simulink model "PMSMpanel_3_1502"  (Simulink 9.2)
settings: Solver=ode45  StartTime=0.0  StopTime=10  RelTol=1e-6  AbsTol=1e-8
values from neighbouring files (symbols this model uses):
  B = 0.08    [PMSMMainprog.m]
  Ba = alpha_s*J_hat - B_hat    (= 1.17)    [PMSMMainprog.m]
  Beta_1 = 113.8*pi/180    (= 1.98618468877)    [PMSMMainprog.m]
  Beta_1_time = 0    [PMSMMainprog.m]
  Beta_2 = 130*pi/180    (= 2.26892802759)    [PMSMMainprog.m]
  Beta_2_time = 2.3    [PMSMMainprog.m]
  Hcd = 1/kpcd    (= 0.0289855072464)    [PMSMMainprog.m]
  Hcq = 1/kpcq    (= 0.0116959064327)    [PMSMMainprog.m]
  i_sd0 = 0*-1.95    (= 0)    [PMSMMainprog.m]
  i_sq0 = 0*4.55    (= 0)    [PMSMMainprog.m]
  iconvlim = 6.5 * sqrt(2)    [PMSMMainprog.m]
  J = 0.0125    [PMSMMainprog.m]
  kicd = alpha_c * (Racd + R_hat)    (= 34500)    [PMSMMainprog.m]
  kicq = alpha_c * (Racq + R_hat)    (= 85500)    [PMSMMainprog.m]
  kis = alpha_s * ( Ba + B_hat)    (= 125)    [PMSMMainprog.m]
  kpcd = alpha_c * L_sd_hat    (= 34.5)    [PMSMMainprog.m]
  kpcq = alpha_c * L_sq_hat    (= 85.5)    [PMSMMainprog.m]
  kps = alpha_s  *J_hat    (= 1.25)    [PMSMMainprog.m]
  L_sd = Laa0 + Lab0 + 1.5 * Laa2    (= 0.0345)    [PMSMMainprog.m]
  L_sd_hat = 0.0345    [PMSMMainprog.m]
  L_sq = Laa0 + Lab0 - 1.5 * Laa2    (= 0.0855)    [PMSMMainprog.m]
  L_sq_hat = 0.0855    [PMSMMainprog.m]
  np = 60 * f/n_s    (= 2)    [PMSMMainprog.m]
  psi_m = 0.822    [PMSMMainprog.m]
  R = 1.33    [PMSMMainprog.m]
  Racd = alpha_c*L_sd_hat - R_hat    (= 33.17)    [PMSMMainprog.m]
  Racq = alpha_c*L_sq_hat - R_hat    (= 84.17)    [PMSMMainprog.m]
  Teref1 = 16.6    [PMSMMainprog.m]
  Teref1_time = 0.1    [PMSMMainprog.m]
  Teref2 = 4    [PMSMMainprog.m]
  Teref2_time = 2.7    [PMSMMainprog.m]
  theta_r0 = 0    [PMSMMainprog.m]
  Tstep = 4    [PMSMMainprog.m]
  Tstep_time = 1.1    [PMSMMainprog.m]
  usd0 = 0*-125    (= 0)    [PMSMMainprog.m]
  usq0 = 0*243    (= 0)    [PMSMMainprog.m]
  VconvLim = 440 * sqrt(2/3)    [PMSMMainprog.m]
  w_r0 = 0*2*pi*50/np    (= 0)    [PMSMMainprog.m]
  wrref = 1500*2*pi/60    (= 157.079632679)    [PMSMMainprog.m]
  wrref_time = 0.1    [PMSMMainprog.m]
  ws = 2*pi*50    (= 314.159265359)    [PMSMMainprog.m]    (also in PostProssPMSM.m = ones(s,1).*ws)
undefined symbols (not defined in the file or in its folder): j
settings Model: Creator=e6zebra  LastModifiedBy=Raghuram  ExtModeTrigMode=oneshot  ExtModeArmWhenConnect=off  ExtModeAutoUpdateStatusClock=off
settings SolverCC: AutoScaleAbsTol=off
settings DataIOCC: LimitDataPoints=off
settings OptimizationCC: BlockReduction=off  BooleanDataType=off  ExpressionDepthLimit=2147483647  InitFltsAndDblsToZero=on
settings DebuggingCC: SaveWithParameterizedLinksMsg=none  SignalResolutionControl=TryResolveAllWithWarning  MultiTaskDSMMsg=warning  MultiTaskCondExecSysMsg=none
settings HardwareCC: TargetUnknown=on
settings RTWCC: TemplateMakefile=grt.tmf
settings GRTTargetCC: TargetFcnLib=ansi_tfl_tmw.mat
settings ConfigComp: CovSFcnEnable=off

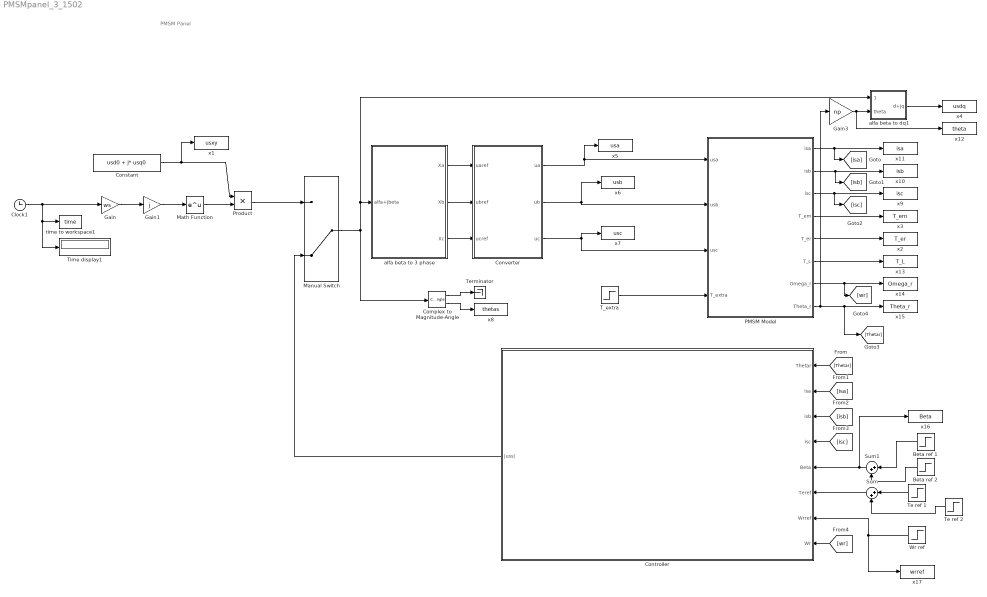
== system PMSMpanel_3_1502 ==
  note: PMSM Panel
  Beta ref 1 : Step  Time=Beta_1_time  After=Beta_1  SampleTime=0
  Beta ref 2 : Step  Time=Beta_2_time  After=Beta_2  SampleTime=0
  Clock1 : Clock
  Complex to Magnitude-Angle : ComplexToMagnitudeAngle
  Constant : Constant  Value=usd0 + j* usq0
  Controller : Subsystem
  Converter : Subsystem
  Gain : Gain  Gain=ws
  Gain1 : Gain  Gain=j
  Gain3 : Gain  Gain=np
  Manual Switch : ManualSwitch  CurrentSetting=0
  Math Function : Math  SaturateOnIntegerOverflow=on
  PMSM Model : Subsystem
  Product : Product
  Sum : Sum  Inputs=|++
  Sum1 : Sum  Inputs=|++
  T_extra : Step  Time=Tstep_time  After=Tstep  SampleTime=0
  Te ref 1 : Step  Time=Teref1_time  After=Teref1  SampleTime=0
  Te ref 2 : Step  Time=Teref2_time  After=Teref2  SampleTime=0
  Terminator : Terminator
  Time display1 : Display
  Wr ref : Step  Time=wrref_time  After=wrref  SampleTime=0
  alfa beta to 3 phase : Subsystem
  alfa beta to dq1 : Subsystem
  time to workspace1 : ToWorkspace  VariableName=time  SampleTime=-1
  x1 : ToWorkspace  VariableName=usxy  SampleTime=-1
  x10 : ToWorkspace  VariableName=isb  SampleTime=-1
  x11 : ToWorkspace  VariableName=isa  SampleTime=-1
  x12 : ToWorkspace  VariableName=theta  SampleTime=-1
  x13 : ToWorkspace  VariableName=T_L  SampleTime=-1
  x14 : ToWorkspace  VariableName=Omega_r  SampleTime=-1
  x15 : ToWorkspace  VariableName=Theta_r  SampleTime=-1
  x16 : ToWorkspace  VariableName=Beta  SampleTime=-1
  x17 : ToWorkspace  VariableName=wrref  SampleTime=-1
  x2 : ToWorkspace  VariableName=T_er  SampleTime=-1
  x3 : ToWorkspace  VariableName=T_em  SampleTime=-1
  x4 : ToWorkspace  VariableName=usdq  SampleTime=-1
  x5 : ToWorkspace  VariableName=usa  SampleTime=-1
  x6 : ToWorkspace  VariableName=usb  SampleTime=-1
  x7 : ToWorkspace  VariableName=usc  SampleTime=-1
  x8 : ToWorkspace  VariableName=thetas  SampleTime=-1
  x9 : ToWorkspace  VariableName=isc  SampleTime=-1
  wires:
  PMSM Model/3(isc) -> [isc], x9/1
  PMSM Model/1(isa) -> [isa], x11/1
  PMSM Model/2(isb) -> [isb], x10/1
  Converter/1(ua) -> x5/1, PMSM Model/1(usa)
  Converter/2(ub) -> x6/1, PMSM Model/2(usb)
  Converter/3(uc) -> PMSM Model/3(usc), x7/1
  T_extra/1 -> PMSM Model/4(T_extra)
  PMSM Model/6(T_L) -> x13/1
  PMSM Model/7(Omega_r) -> [wr], x14/1
  PMSM Model/5(T_er) -> x2/1
  PMSM Model/4(T_em) -> x3/1
  Gain1/1 -> Math Function/1
  Gain/1 -> Gain1/1
  Math Function/1 -> Product/2
  Constant/1 -> Product/1, x1/1
  Clock1/1 -> Time display1/1, time to workspace1/1, Gain/1
  Manual Switch/1 -> Complex to Magnitude-Angle/1, alfa beta to dq1/1(alfa+jbeta), alfa beta to 3 phase/1(alfa+jbeta)
  alfa beta to 3 phase/1(Xa) -> Converter/1(uaref)
  alfa beta to 3 phase/2(Xb) -> Converter/2(ubref)
  alfa beta to 3 phase/3(Xc) -> Converter/3(ucref)
  alfa beta to dq1/1(d+jq) -> x4/1
  Complex to Magnitude-Angle/1 -> Terminator/1
  Complex to Magnitude-Angle/2 -> x8/1
  PMSM Model/8(Theta_r) -> [Thetar], x15/1, Gain3/1
  Gain3/1 -> x12/1, alfa beta to dq1/2(theta)
  Product/1 -> Manual Switch/1
  [Thetar] -> Controller/1(Thetar)
  [isa] -> Controller/2(isa)
  [isb] -> Controller/3(isb)
  [isc] -> Controller/4(isc)
  Wr ref/1 -> Controller/7(Wrref), x17/1
  Controller/1(|uss|) -> Manual Switch/2
  [wr] -> Controller/8(Wr)
  Te ref 2/1 -> Sum/2
  Te ref 1/1 -> Sum/1
  Sum/1 -> Controller/6(Teref)
  Beta ref 1/1 -> Sum1/1
  Beta ref 2/1 -> Sum1/2
  Sum1/1 -> Controller/5(Beta), x16/1

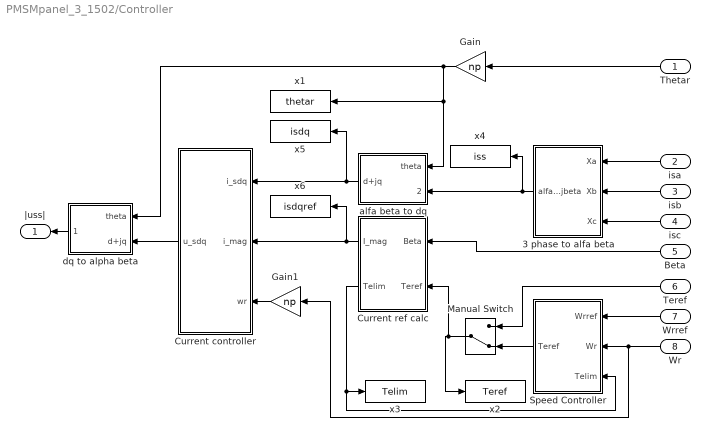
== system PMSMpanel_3_1502/Controller ==
  Thetar : Inport
  isa : Inport  Port=2
  isb : Inport  Port=3
  isc : Inport  Port=4
  Beta : Inport  Port=5
  Teref : Inport  Port=6
  Wrref : Inport  Port=7
  Wr : Inport  Port=8
  3 phase to alfa beta : Subsystem
  Current controller : Subsystem
  Current ref calc : Subsystem
  Gain : Gain  Gain=np
  Gain1 : Gain  Gain=np
  Manual Switch : ManualSwitch  CurrentSetting=0
  Speed Controller : Subsystem
  alfa beta to dq : Subsystem
  dq to alpha beta : Subsystem
  x1 : ToWorkspace  VariableName=thetar  SampleTime=-1
  x2 : ToWorkspace  VariableName=Teref  SampleTime=-1
  x3 : ToWorkspace  VariableName=Telim  SampleTime=-1
  x4 : ToWorkspace  VariableName=iss  SampleTime=-1
  x5 : ToWorkspace  VariableName=isdq  SampleTime=-1
  x6 : ToWorkspace  VariableName=isdqref  SampleTime=-1
  |uss| : Outport
  wires:
  isa/1 -> 3 phase to alfa beta/1(Xa)
  isb/1 -> 3 phase to alfa beta/2(Xb)
  isc/1 -> 3 phase to alfa beta/3(Xc)
  Thetar/1 -> Gain/1
  3 phase to alfa beta/1(alfa+jbeta) -> alfa beta to dq/2(alfa+jbeta), x4/1
  Gain/1 -> x1/1, alfa beta to dq/1(theta), dq to alpha beta/1(theta)
  dq to alpha beta/1(alfa+jbeta) -> |uss|/1
  Wrref/1 -> Speed Controller/1(Wrref)
  Wr/1 -> Gain1/1, Speed Controller/2(Wr)
  Teref/1 -> Manual Switch/1
  Speed Controller/1(Teref) -> Manual Switch/2
  Beta/1 -> Current ref calc/1(Beta)
  Manual Switch/1 -> Current ref calc/2(Teref), x2/1
  Gain1/1 -> Current controller/3(wr)
  Current ref calc/2(Telim) -> x3/1, Speed Controller/3(Telim)
  alfa beta to dq/1(d+jq) -> x5/1, Current controller/1(i_sdq)
  Current controller/1(u_sdq) -> dq to alpha beta/2(d+jq)
  Current ref calc/1(I_mag) -> Current controller/2(i_mag), x6/1

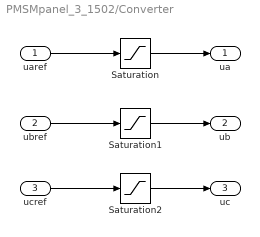
== system PMSMpanel_3_1502/Converter ==
  uaref : Inport
  ubref : Inport  Port=2
  ucref : Inport  Port=3
  Saturation : Saturate  UpperLimit=VconvLim  LowerLimit=-VconvLim
  Saturation1 : Saturate  UpperLimit=VconvLim  LowerLimit=-VconvLim
  Saturation2 : Saturate  UpperLimit=VconvLim  LowerLimit=-VconvLim
  ua : Outport
  ub : Outport  Port=2
  uc : Outport  Port=3
  wires:
  Saturation2/1 -> uc/1
  Saturation1/1 -> ub/1
  Saturation/1 -> ua/1
  uaref/1 -> Saturation/1
  ubref/1 -> Saturation1/1
  ucref/1 -> Saturation2/1

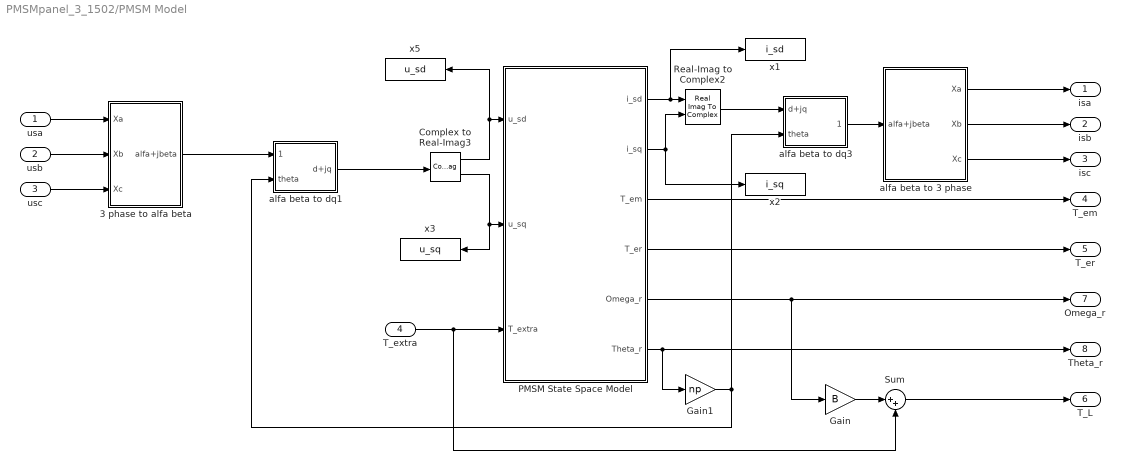
== system PMSMpanel_3_1502/PMSM Model ==
  usa : Inport
  usb : Inport  Port=2
  usc : Inport  Port=3
  T_extra : Inport  Port=4
  3 phase to alfa beta : Subsystem
  Complex to Real-Imag3 : ComplexToRealImag
  Gain : Gain  Gain=B
  Gain1 : Gain  Gain=np
  PMSM State Space Model : Subsystem
  Real-Imag to Complex2 : RealImagToComplex
  Sum : Sum  Inputs=|++
  alfa beta to 3 phase : Subsystem
  alfa beta to dq1 : Subsystem
  alfa beta to dq3 : Subsystem
  x1 : ToWorkspace  VariableName=i_sd  SampleTime=-1
  x2 : ToWorkspace  VariableName=i_sq  SampleTime=-1
  x3 : ToWorkspace  VariableName=u_sq  SampleTime=-1
  x5 : ToWorkspace  VariableName=u_sd  SampleTime=-1
  isa : Outport
  isb : Outport  Port=2
  isc : Outport  Port=3
  T_em : Outport  Port=4
  T_er : Outport  Port=5
  T_L : Outport  Port=6
  Omega_r : Outport  Port=7
  Theta_r : Outport  Port=8
  wires:
  3 phase to alfa beta/1(alfa+jbeta) -> alfa beta to dq1/1(alfa+jbeta)
  alfa beta to dq1/1(d+jq) -> Complex to Real-Imag3/1
  usb/1 -> 3 phase to alfa beta/2(Xb)
  usc/1 -> 3 phase to alfa beta/3(Xc)
  usa/1 -> 3 phase to alfa beta/1(Xa)
  alfa beta to 3 phase/1(Xa) -> isa/1
  alfa beta to 3 phase/2(Xb) -> isb/1
  alfa beta to 3 phase/3(Xc) -> isc/1
  Real-Imag to Complex2/1 -> alfa beta to dq3/1(d+jq)
  alfa beta to dq3/1(alfa+jbeta) -> alfa beta to 3 phase/1(alfa+jbeta)
  T_extra/1 -> PMSM State Space Model/3(T_extra), Sum/2
  Gain/1 -> Sum/1
  Sum/1 -> T_L/1
  Gain1/1 -> alfa beta to dq3/2(theta), alfa beta to dq1/2(theta)
  Complex to Real-Imag3/2 -> x3/1, PMSM State Space Model/2(u_sq)
  Complex to Real-Imag3/1 -> PMSM State Space Model/1(u_sd), x5/1
  PMSM State Space Model/1(i_sd) -> x1/1, Real-Imag to Complex2/1
  PMSM State Space Model/2(i_sq) -> x2/1, Real-Imag to Complex2/2
  PMSM State Space Model/6(Theta_r) -> Gain1/1, Theta_r/1
  PMSM State Space Model/5(Omega_r) -> Gain/1, Omega_r/1
  PMSM State Space Model/4(T_er) -> T_er/1
  PMSM State Space Model/3(T_em) -> T_em/1

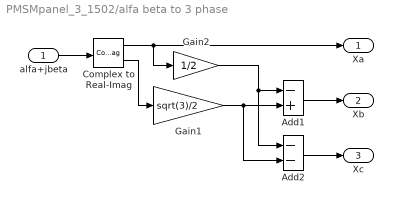
== system PMSMpanel_3_1502/alfa beta to 3 phase ==
  alfa+jbeta : Inport
  Add1 : Sum  Inputs=-+
  Add2 : Sum  Inputs=--
  Complex to Real-Imag : ComplexToRealImag
  Gain1 : Gain  Gain=sqrt(3)/2
  Gain2 : Gain  Gain=1/2
  Xa : Outport
  Xb : Outport  Port=2
  Xc : Outport  Port=3
  wires:
  alfa+jbeta/1 -> Complex to Real-Imag/1
  Complex to Real-Imag/1 -> Xa/1, Gain2/1
  Add2/1 -> Xc/1
  Add1/1 -> Xb/1
  Complex to Real-Imag/2 -> Gain1/1
  Gain1/1 -> Add1/2, Add2/2
  Gain2/1 -> Add1/1, Add2/1

== system PMSMpanel_3_1502/alfa beta to dq1 ==
  alfa+jbeta : Inport
  theta : Inport  Port=2
  Gain : Gain  Gain=-j  SaturateOnIntegerOverflow=on  OutDataTypeStr=Inherit: Same as input  ParamDataTypeStr=Inherit: Same as input
  Math Function : Math  SaturateOnIntegerOverflow=on
  Product : Product  SaturateOnIntegerOverflow=on  OutDataTypeStr=Inherit: Same as first input
  d+jq : Outport
  wires:
  theta/1 -> Gain/1
  Gain/1 -> Math Function/1
  Math Function/1 -> Product/2
  alfa+jbeta/1 -> Product/1
  Product/1 -> d+jq/1

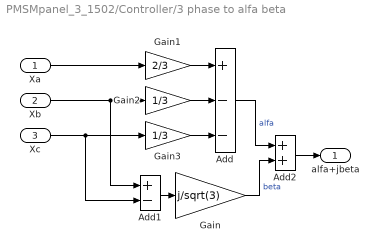
== system PMSMpanel_3_1502/Controller/3 phase to alfa beta ==
  Xa : Inport
  Xb : Inport  Port=2
  Xc : Inport  Port=3
  Add : Sum  Inputs=+--
  Add1 : Sum  Inputs=+-
  Add2 : Sum
  Gain : Gain  Gain=j/sqrt(3)
  Gain1 : Gain  Gain=2/3
  Gain2 : Gain  Gain=1/3
  Gain3 : Gain  Gain=1/3
  alfa+jbeta : Outport
  wires:
  Add1/1 -> Gain/1
  Add2/1 -> alfa+jbeta/1
  Gain/1 -> Add2/2  "beta"
  Add/1 -> Add2/1  "alfa"
  Gain3/1 -> Add/3
  Gain2/1 -> Add/2
  Gain1/1 -> Add/1
  Xa/1 -> Gain1/1
  Xb/1 -> Gain2/1, Add1/1
  Xc/1 -> Gain3/1, Add1/2

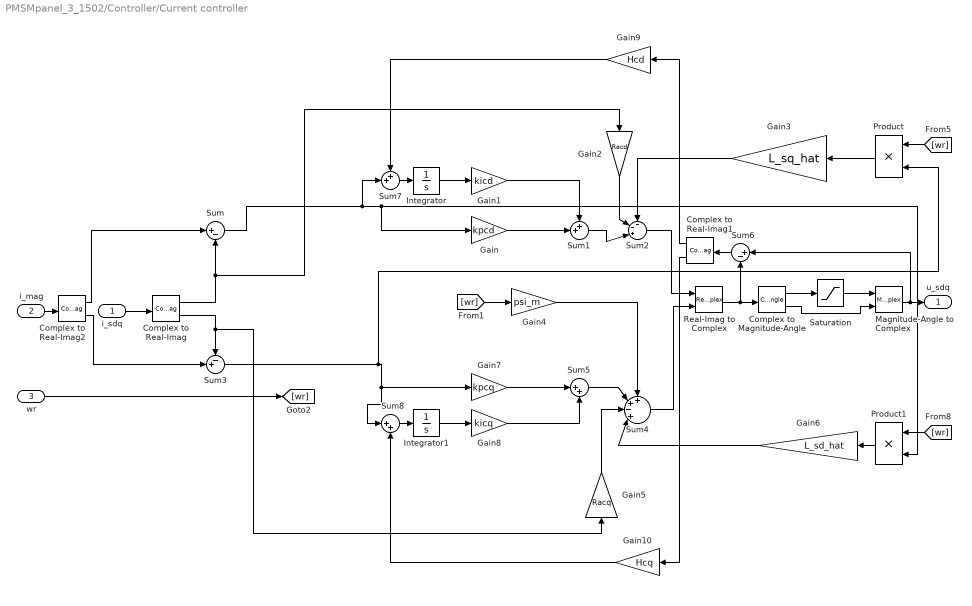
== system PMSMpanel_3_1502/Controller/Current controller ==
  i_sdq : Inport
  i_mag : Inport  Port=2
  wr : Inport  Port=3
  Complex to Magnitude-Angle : ComplexToMagnitudeAngle
  Complex to Real-Imag : ComplexToRealImag
  Complex to Real-Imag1 : ComplexToRealImag
  Complex to Real-Imag2 : ComplexToRealImag
  Gain : Gain  Gain=kpcd
  Gain1 : Gain  Gain=kicd
  Gain10 : Gain  Gain=Hcq
  Gain2 : Gain  Gain=Racd
  Gain3 : Gain  Gain=L_sq_hat
  Gain4 : Gain  Gain=psi_m
  Gain5 : Gain  Gain=Racq
  Gain6 : Gain  Gain=L_sd_hat
  Gain7 : Gain  Gain=kpcq
  Gain8 : Gain  Gain=kicq
  Gain9 : Gain  Gain=Hcd
  Integrator : Integrator  InitialCondition=i_sd0
  Integrator1 : Integrator  InitialCondition=i_sq0
  Magnitude-Angle to Complex : MagnitudeAngleToComplex
  Product : Product
  Product1 : Product
  Real-Imag to Complex : RealImagToComplex
  Saturation : Saturate  UpperLimit=VconvLim  LowerLimit=-VconvLim
  Sum : Sum  Inputs=|+-
  Sum1 : Sum  Inputs=++|
  Sum2 : Sum  Inputs=--+|
  Sum3 : Sum  Inputs=-+|
  Sum4 : Sum  Inputs=++-+|
  Sum5 : Sum  Inputs=|++
  Sum6 : Sum  Inputs=|+-
  Sum7 : Sum  Inputs=++|
  Sum8 : Sum  Inputs=|++
  u_sdq : Outport
  wires:
  wr/1 -> [wr]
  Gain/1 -> Sum1/2
  Gain1/1 -> Sum1/1
  Integrator/1 -> Gain1/1
  Sum1/1 -> Sum2/3
  Complex to Real-Imag/1 -> Gain2/1, Sum/2
  Gain2/1 -> Sum2/2
  [wr] -> Product/1
  Sum3/1 -> Product/2, Sum8/1, Gain7/1
  Product/1 -> Gain3/1
  Gain3/1 -> Sum2/1
  Sum2/1 -> Real-Imag to Complex/1
  [wr] -> Gain4/1
  i_sdq/1 -> Complex to Real-Imag/1
  Gain4/1 -> Sum4/1
  Complex to Real-Imag/2 -> Gain5/1, Sum3/1
  Gain5/1 -> Sum4/3
  Product1/1 -> Gain6/1
  Sum/1 -> Product1/2, Gain/1, Sum7/2
  [wr] -> Product1/1
  Gain6/1 -> Sum4/4
  Sum4/1 -> Real-Imag to Complex/2
  Integrator1/1 -> Gain8/1
  Gain8/1 -> Sum5/2
  Gain7/1 -> Sum5/1
  Sum5/1 -> Sum4/2
  Real-Imag to Complex/1 -> Sum6/2, Complex to Magnitude-Angle/1
  Complex to Magnitude-Angle/1 -> Saturation/1
  Saturation/1 -> Magnitude-Angle to Complex/1
  Complex to Magnitude-Angle/2 -> Magnitude-Angle to Complex/2
  Magnitude-Angle to Complex/1 -> Sum6/1, u_sdq/1
  Sum6/1 -> Complex to Real-Imag1/1
  Complex to Real-Imag1/2 -> Gain10/1
  Complex to Real-Imag1/1 -> Gain9/1
  Sum7/1 -> Integrator/1
  Gain9/1 -> Sum7/1
  Sum8/1 -> Integrator1/1
  Gain10/1 -> Sum8/2
  i_mag/1 -> Complex to Real-Imag2/1
  Complex to Real-Imag2/1 -> Sum/1
  Complex to Real-Imag2/2 -> Sum3/2

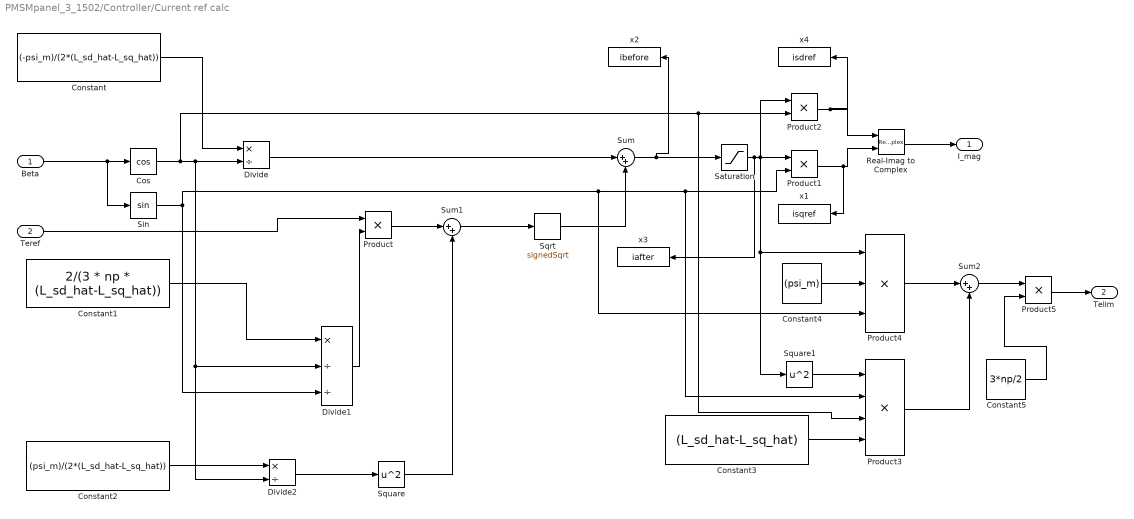
== system PMSMpanel_3_1502/Controller/Current ref calc ==
  Beta : Inport
  Teref : Inport  Port=2
  Constant : Constant  Value=(-psi_m)/(2*(L_sd_hat-L_sq_hat))
  Constant1 : Constant  Value=2/(3 * np * (L_sd_hat-L_sq_hat))
  Constant2 : Constant  Value=(psi_m)/(2*(L_sd_hat-L_sq_hat))
  Constant3 : Constant  Value=(L_sd_hat-L_sq_hat)
  Constant4 : Constant  Value=(psi_m)
  Constant5 : Constant  Value=3*np/2
  Cos : Trigonometry  Operator=cos
  Divide : Product  Inputs=*/
  Divide1 : Product  Inputs=*//
  Divide2 : Product  Inputs=*/
  Product{,1..2,5} (4 alike) : Product
  Product3 : Product  Inputs=4
  Product4 : Product  Inputs=3
  Real-Imag to Complex : RealImagToComplex
  Saturation : Saturate  UpperLimit=iconvlim  LowerLimit=-iconvlim
  Sin : Trigonometry
  Sqrt : Sqrt  Operator=signedSqrt  SaturateOnIntegerOverflow=on
  Square : Math  Operator=square  SaturateOnIntegerOverflow=on
  Square1 : Math  Operator=square  SaturateOnIntegerOverflow=on
  Sum : Sum  Inputs=|++
  Sum1 : Sum  Inputs=|++
  Sum2 : Sum  Inputs=|++
  x1 : ToWorkspace  VariableName=isqref  SampleTime=-1
  x2 : ToWorkspace  VariableName=ibefore  SampleTime=-1
  x3 : ToWorkspace  VariableName=iafter  SampleTime=-1
  x4 : ToWorkspace  VariableName=isdref  SampleTime=-1
  I_mag : Outport  VectorParamsAs1DForOutWhenUnconnected=on
  Telim : Outport  Port=2  VectorParamsAs1DForOutWhenUnconnected=on
  wires:
  Beta/1 -> Sin/1, Cos/1
  Cos/1 -> Product3/3, Product2/2, Divide2/2, Divide1/2, Divide/2
  Constant/1 -> Divide/1
  Divide/1 -> Sum/1
  Constant1/1 -> Divide1/1
  Sin/1 -> Divide1/3, Product4/3, Product3/2, Product1/2
  Divide1/1 -> Product/2
  Teref/1 -> Product/1
  Product/1 -> Sum1/1
  Constant2/1 -> Divide2/1
  Divide2/1 -> Square/1
  Square/1 -> Sum1/2
  Sum1/1 -> Sqrt/1
  Sqrt/1 -> Sum/2
  Saturation/1 -> x3/1, Product4/1, Square1/1, Product2/1, Product1/1
  Product2/1 -> x4/1, Real-Imag to Complex/1
  Product1/1 -> x1/1, Real-Imag to Complex/2
  Real-Imag to Complex/1 -> I_mag/1
  Square1/1 -> Product3/1
  Constant3/1 -> Product3/4
  Constant4/1 -> Product4/2
  Product4/1 -> Sum2/1
  Product3/1 -> Sum2/2
  Sum2/1 -> Product5/1
  Constant5/1 -> Product5/2
  Product5/1 -> Telim/1
  Sum/1 -> x2/1, Saturation/1

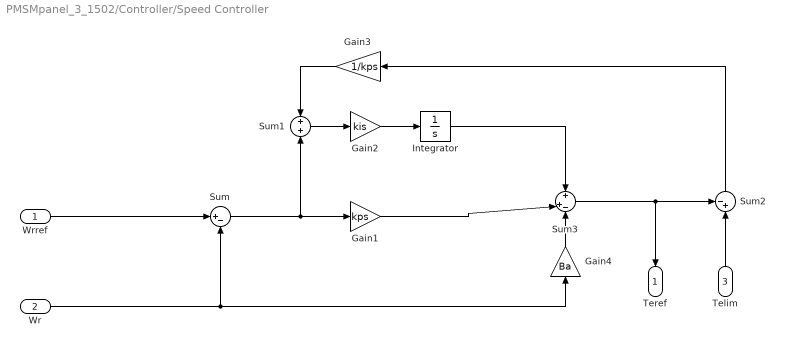
== system PMSMpanel_3_1502/Controller/Speed Controller ==
  Wrref : Inport
  Wr : Inport  Port=2
  Telim : Inport  Port=3
  Gain1 : Gain  Gain=kps
  Gain2 : Gain  Gain=kis
  Gain3 : Gain  Gain=1/kps
  Gain4 : Gain  Gain=Ba
  Integrator : Integrator
  Sum : Sum  Inputs=|+-
  Sum1 : Sum  Inputs=+|+
  Sum2 : Sum  Inputs=-+|
  Sum3 : Sum  Inputs=+|+-
  Teref : Outport
  wires:
  Sum1/1 -> Gain2/1
  Gain2/1 -> Integrator/1
  Gain3/1 -> Sum1/1
  Integrator/1 -> Sum3/1
  Sum/1 -> Gain1/1, Sum1/2
  Wrref/1 -> Sum/1
  Wr/1 -> Sum/2, Gain4/1
  Gain4/1 -> Sum3/3
  Gain1/1 -> Sum3/2
  Sum3/1 -> Teref/1, Sum2/1
  Telim/1 -> Sum2/2
  Sum2/1 -> Gain3/1

== system PMSMpanel_3_1502/Controller/alfa beta to dq ==
  theta : Inport
  alfa+jbeta : Inport  Port=2
  Gain : Gain  Gain=-j  SaturateOnIntegerOverflow=on  OutDataTypeStr=Inherit: Same as input  ParamDataTypeStr=Inherit: Same as input
  Math Function : Math  SaturateOnIntegerOverflow=on
  Product : Product  SaturateOnIntegerOverflow=on  OutDataTypeStr=Inherit: Same as first input
  d+jq : Outport
  wires:
  theta/1 -> Gain/1
  Gain/1 -> Math Function/1
  Math Function/1 -> Product/2
  alfa+jbeta/1 -> Product/1
  Product/1 -> d+jq/1

== system PMSMpanel_3_1502/Controller/dq to alpha beta ==
  theta : Inport
  d+jq : Inport  Port=2
  Gain : Gain  Gain=j  SaturateOnIntegerOverflow=on  OutDataTypeStr=Inherit: Same as input  ParamDataTypeStr=Inherit: Same as input
  Math Function : Math  SaturateOnIntegerOverflow=on
  Product : Product  SaturateOnIntegerOverflow=on  OutDataTypeStr=Inherit: Same as first input
  alfa+jbeta : Outport
  wires:
  Product/1 -> alfa+jbeta/1
  d+jq/1 -> Product/1
  Math Function/1 -> Product/2
  Gain/1 -> Math Function/1
  theta/1 -> Gain/1

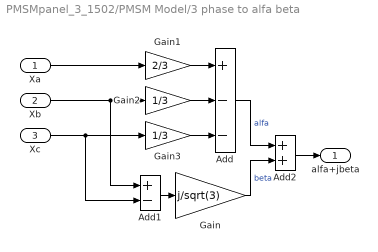
== system PMSMpanel_3_1502/PMSM Model/3 phase to alfa beta ==
  Xa : Inport
  Xb : Inport  Port=2
  Xc : Inport  Port=3
  Add : Sum  Inputs=+--
  Add1 : Sum  Inputs=+-
  Add2 : Sum
  Gain : Gain  Gain=j/sqrt(3)
  Gain1 : Gain  Gain=2/3
  Gain2 : Gain  Gain=1/3
  Gain3 : Gain  Gain=1/3
  alfa+jbeta : Outport
  wires:
  Add1/1 -> Gain/1
  Add2/1 -> alfa+jbeta/1
  Gain/1 -> Add2/2  "beta"
  Add/1 -> Add2/1  "alfa"
  Gain3/1 -> Add/3
  Gain2/1 -> Add/2
  Gain1/1 -> Add/1
  Xa/1 -> Gain1/1
  Xb/1 -> Gain2/1, Add1/1
  Xc/1 -> Gain3/1, Add1/2

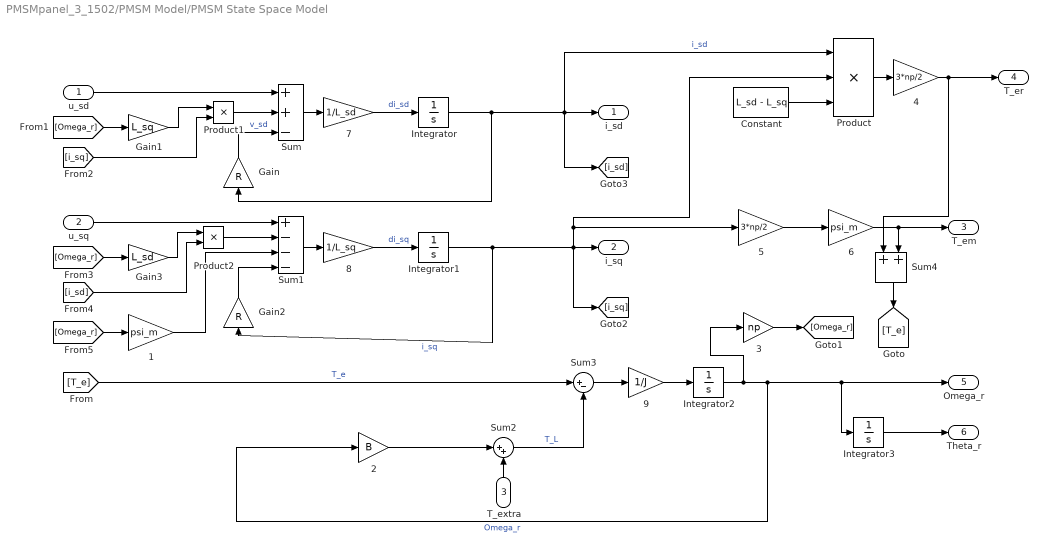
== system PMSMpanel_3_1502/PMSM Model/PMSM State Space Model ==
  u_sd : Inport
  u_sq : Inport  Port=2
  T_extra : Inport  Port=3
  "  1" : Gain  Gain=psi_m
  "  2" : Gain  Gain=B
  "  3" : Gain  Gain=np
  "  4" : Gain  Gain=3*np/2
  "  5" : Gain  Gain=3*np/2
  "  6" : Gain  Gain=psi_m
  "  7" : Gain  Gain=1/L_sd
  "  8" : Gain  Gain=1/L_sq
  "  9" : Gain  Gain=1/J
  Constant : Constant  Value=L_sd - L_sq
  Gain : Gain  Gain=R
  Gain1 : Gain  Gain=L_sq
  Gain2 : Gain  Gain=R
  Gain3 : Gain  Gain=L_sd
  Integrator : Integrator  InitialCondition=i_sd0
  Integrator1 : Integrator  InitialCondition=i_sq0
  Integrator2 : Integrator  InitialCondition=w_r0
  Integrator3 : Integrator  InitialCondition=theta_r0
  Product : Product  Inputs=3
  Product1 : Product
  Product2 : Product
  Sum : Sum  Inputs=++-
  Sum1 : Sum  Inputs=+---
  Sum2 : Sum  Inputs=|++
  Sum3 : Sum  Inputs=|+-
  Sum4 : Sum
  i_sd : Outport
  i_sq : Outport  Port=2
  T_em : Outport  Port=3
  T_er : Outport  Port=4
  Omega_r : Outport  Port=5
  Theta_r : Outport  Port=6
  wires:
  "  8"/1 -> Integrator1/1  "di_sq"
  Sum1/1 -> "  8"/1
  Integrator1/1 -> Gain2/1, Product/2, "  5"/1, i_sq/1, [i_sq]  "i_sq"
  u_sq/1 -> Sum1/1
  Integrator/1 -> Gain/1, i_sd/1, [i_sd], Product/1  "i_sd"
  "  7"/1 -> Integrator/1  "di_sd"
  Sum/1 -> "  7"/1
  u_sd/1 -> Sum/1
  T_extra/1 -> Sum2/2
  "  2"/1 -> Sum2/1
  "  5"/1 -> "  6"/1
  "  6"/1 -> T_em/1, Sum4/2
  Constant/1 -> Product/3
  Product/1 -> "  4"/1
  Sum2/1 -> Sum3/2  "T_L"
  Sum4/1 -> [T_e]
  [T_e] -> Sum3/1  "T_e"
  Sum3/1 -> "  9"/1
  "  9"/1 -> Integrator2/1
  Integrator2/1 -> "  3"/1, Integrator3/1, Omega_r/1, "  2"/1  "Omega_r"
  Integrator3/1 -> Theta_r/1
  Gain/1 -> Sum/3  "v_sd"
  [Omega_r] -> Gain1/1
  Gain1/1 -> Product1/1
  Product1/1 -> Sum/2
  [i_sq] -> Product1/2
  [i_sd] -> Product2/2
  Gain3/1 -> Product2/1
  [Omega_r] -> Gain3/1
  Product2/1 -> Sum1/2
  Gain2/1 -> Sum1/4
  [Omega_r] -> "  1"/1
  "  1"/1 -> Sum1/3
  "  3"/1 -> [Omega_r]
  "  4"/1 -> T_er/1, Sum4/1

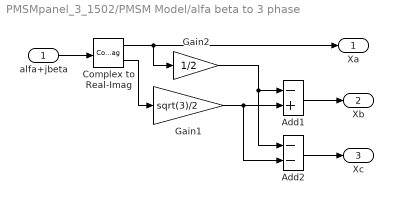
== system PMSMpanel_3_1502/PMSM Model/alfa beta to 3 phase ==
  alfa+jbeta : Inport
  Add1 : Sum  Inputs=-+
  Add2 : Sum  Inputs=--
  Complex to Real-Imag : ComplexToRealImag
  Gain1 : Gain  Gain=sqrt(3)/2
  Gain2 : Gain  Gain=1/2
  Xa : Outport
  Xb : Outport  Port=2
  Xc : Outport  Port=3
  wires:
  alfa+jbeta/1 -> Complex to Real-Imag/1
  Complex to Real-Imag/1 -> Xa/1, Gain2/1
  Add2/1 -> Xc/1
  Add1/1 -> Xb/1
  Complex to Real-Imag/2 -> Gain1/1
  Gain1/1 -> Add1/2, Add2/2
  Gain2/1 -> Add1/1, Add2/1

== system PMSMpanel_3_1502/PMSM Model/alfa beta to dq1 ==
  alfa+jbeta : Inport
  theta : Inport  Port=2
  Gain : Gain  Gain=-j  SaturateOnIntegerOverflow=on  OutDataTypeStr=Inherit: Same as input  ParamDataTypeStr=Inherit: Same as input
  Math Function : Math  SaturateOnIntegerOverflow=on
  Product : Product  SaturateOnIntegerOverflow=on  OutDataTypeStr=Inherit: Same as first input
  d+jq : Outport
  wires:
  theta/1 -> Gain/1
  Gain/1 -> Math Function/1
  Math Function/1 -> Product/2
  alfa+jbeta/1 -> Product/1
  Product/1 -> d+jq/1

== system PMSMpanel_3_1502/PMSM Model/alfa beta to dq3 ==
  d+jq : Inport
  theta : Inport  Port=2
  Gain : Gain  Gain=j  SaturateOnIntegerOverflow=on  OutDataTypeStr=Inherit: Same as input  ParamDataTypeStr=Inherit: Same as input
  Math Function : Math  SaturateOnIntegerOverflow=on
  Product : Product  SaturateOnIntegerOverflow=on  OutDataTypeStr=Inherit: Same as first input
  alfa+jbeta : Outport
  wires:
  Product/1 -> alfa+jbeta/1
  d+jq/1 -> Product/1
  Math Function/1 -> Product/2
  Gain/1 -> Math Function/1
  theta/1 -> Gain/1
